simulink model "rlDDPG4PFC2"  (R2022b)
settings: Solver=FixedStepAuto  StartTime=0.0  StopTime=Tf  FixedStep=0.001  RelTol=1e-3
StartFcn:
  | %scopes= find_system(bdroot,'BlockType','Scope');
  | %for i = 1:length(scopes)
  | %set_param(scopes{i},'Open','on');
  | %end
values from neighbouring files (symbols this model uses):
  amax_ego = 0.4    [DDPG_1.m]    (also in DQN4.m)
  amin_ego = -0.5    [DDPG_1.m]    (also in DQN4.m)
  Cf = 19000    [DDPG_1.m]    (also in DQN4.m)
  Cr = 33000    [DDPG_1.m]    (also in DQN4.m)
  D_default = 1.5    [DDPG_1.m]    (also in DQN4.m)
  e1_initial = -0.05    [DDPG_1.m]    (also in DQN4.m)
  e2_initial = 0.05    [DDPG_1.m]    (also in DQN4.m)
  Iz = 2875    [DDPG_1.m]    (also in DQN4.m)
  lf = 1.4    [DDPG_1.m]    (also in DQN4.m)
  lr = 1.6    [DDPG_1.m]    (also in DQN4.m)
  m = 1600    [DDPG_1.m]    (also in DQN4.m)
  t_gap = 1.4    [DDPG_1.m]    (also in DQN4.m)
  target = 1    [DDPG_1.m]    (also in DQN4.m = 3)
  tau = 0.5    [DDPG_1.m]    (also in DQN4.m)
  Ts = 0.1    [DDPG_1.m]    (also in DQN4.m)
  umax_ego = 0.2618    [DDPG_1.m]    (also in DQN4.m)
  umin_ego = -0.2618    [DDPG_1.m]    (also in DQN4.m)
  v0_FV1 = 0.5    [DDPG_1.m]    (also in DQN4.m)
  v0_FV2 = 0.5    [DDPG_1.m]    (also in DQN4.m)
  v0_LV = 0.9    [DDPG_1.m]    (also in DQN4.m)
  v_set = 1.5    [DDPG_1.m]    (also in DQN4.m)
  x0_FV1 = 1.5    [DDPG_1.m]    (also in DQN4.m)
  x0_FV2 = 0    [DDPG_1.m]    (also in DQN4.m)
  x0_LV = 3    [DDPG_1.m]    (also in DQN4.m)
undefined symbols (not defined in the file or in its folder): DiscIntNeverNeededParam, Speed, SteeringAngle
libraries: simulink x19, rllib x4, robotlib x4, dsparch4 x2
(part 2 of 2)

== system rlDDPG4PFC2/Ego Vehicle and Environment3/Lead vehicle1/ramp1 ==
  note: 工况1：斜坡加速度
  Clock : Clock
  Constant1 : Constant  Value=20
  Constant2 : Constant  Value=40
  Ramp : simulink/Sources/Ramp  slope=0.001  start=0  InitialOutput=0
  Ramp1 : simulink/Sources/Ramp  slope=-0.001  start=20  InitialOutput=0.02
  Ramp2 : simulink/Sources/Ramp  slope=0  start=40  InitialOutput=0
  Relational Operator : RelationalOperator  Operator=<=  OutDataTypeStr=boolean  RndMeth=Simplest  InputSameDT=off
  Relational Operator1 : RelationalOperator  Operator=<=  OutDataTypeStr=boolean  RndMeth=Simplest  InputSameDT=off
  Switch : Switch  Criteria=u2 > Threshold  SaturateOnIntegerOverflow=off  InputSameDT=off
  Switch1 : Switch  Criteria=u2 > Threshold  SaturateOnIntegerOverflow=off  InputSameDT=off
  Out1 : Outport
  wires:
  Constant1/1 -> Relational Operator/2
  Ramp1/1 -> Switch1/1
  Relational Operator/1 -> Switch/2
  Switch1/1 -> Switch/3
  Relational Operator1/1 -> Switch1/2
  Clock/1 -> Relational Operator1/1, Relational Operator/1
  Ramp/1 -> Switch/1
  Constant2/1 -> Relational Operator1/2
  Ramp2/1 -> Switch1/3
  Switch/1 -> Out1/1

== system rlDDPG4PFC2/Ego Vehicle and Environment3/Lead vehicle1/step1 ==
  note: 工况3：阶梯式加速-减速
  Add : Sum  Inputs=++++
  Step : Step  Time=5  After=0.2  SampleTime=0
  Step1 : Step  Time=8  After=-0.2  SampleTime=0
  Step2 : Step  Time=40  After=-0.2  SampleTime=0
  Step3 : Step  Time=43  After=0.2  SampleTime=0
  a_LV : Outport
  wires:
  Step2/1 -> Add/3
  Step3/1 -> Add/4
  Step/1 -> Add/1
  Add/1 -> a_LV/1  "a_LV"
  Step1/1 -> Add/2

== matlab function rlDDPG4PFC2/Ego Vehicle and Environment1/curvature1/N-curve ==
  data: s input; rho output
function rho = fcn(s)
% 根据输入s计算输出rho
if s >= 0 && s < 5
  rho = 0;
elseif s >= 5 && s < 10
  rho = 0.025*4;
elseif s >= 10 && s < 30
  rho = -0.025;
elseif s >= 30 && s < 40
  rho = -0.0855;
elseif s >= 40 && s < 60
  rho = 0.057;
else  % s >= 60
  rho = 0;
end

== matlab function rlDDPG4PFC2/Ego Vehicle and Environment1/curvature1/S-curve ==
  data: s input; rho output
function rho = fcn(s)
% 根据输入s计算输出rho
if s >= 0 && s < 10
  rho = 0;
elseif s >= 10 && s < 40
  rho = 0.005*4;
elseif s >= 40 && s < 70
  rho = -0.005*4;
else  % s >= 70
  rho = 0;
end

== matlab function rlDDPG4PFC2/Ego Vehicle and Environment3/curvature1/M-curve ==
  data: s input; rho output
function rho = fcn(s)
% 根据输入s计算输出rho
if s >= 0 && s < 5
  rho = 0;
elseif s >= 5 && s < 13
  rho = 0.1;
elseif s >= 13 && s < 25
  rho = -0.0667;
elseif s >= 25 && s < 27
  rho = 0;
elseif s >= 27 && s < 33
  rho = -0.05;
elseif s >= 33 && s < 53
  rho = 0.03;
elseif s >= 53 && s < 59
    rho = -0.05;
elseif s >= 59 && s < 61
    rho = 0;
elseif s >= 61 && s < 73
  rho = -0.0667;
elseif s >= 73 && s < 81
  rho = 0.1;
else  % s >= 70
  rho = 0;
end

== matlab function rlDDPG4PFC2/Ego Vehicle and Environment3/curvature1/N-curve ==
  data: s input; rho output
function rho = fcn(s)
% 根据输入s计算输出rho
if s >= 0 && s < 5
  rho = 0;
elseif s >= 5 && s < 10
  rho = 0.025*4;
elseif s >= 10 && s < 30
  rho = -0.025;
elseif s >= 30 && s < 40
  rho = -0.0855;
elseif s >= 40 && s < 60
  rho = 0.057;
else  % s >= 60
  rho = 0;
end

== matlab function rlDDPG4PFC2/Ego Vehicle and Environment3/curvature1/S-curve ==
  data: s input; rho output
function rho = fcn(s)
% 根据输入s计算输出rho
if s >= 0 && s < 10
  rho = 0;
elseif s >= 10 && s < 40
  rho = 0.005*4;
elseif s >= 40 && s < 70
  rho = -0.005*4;
else  % s >= 70
  rho = 0;
end

== matlab function rlDDPG4PFC2/Ego Vehicle and Environment1/curvature1/M-curve ==
  data: s input; rho output
function rho = fcn(s)
% 根据输入s计算输出rho
if s >= 0 && s < 5
  rho = 0;
elseif s >= 5 && s < 13
  rho = 0.1;
elseif s >= 13 && s < 25
  rho = -0.0667;
elseif s >= 25 && s < 27
  rho = 0;
elseif s >= 27 && s < 33
  rho = -0.05;
elseif s >= 33 && s < 53
  rho = 0.03;
elseif s >= 53 && s < 59
    rho = -0.05;
elseif s >= 59 && s < 61
    rho = 0;
elseif s >= 61 && s < 73
  rho = -0.0667;
elseif s >= 73 && s < 81
  rho = 0.1;
else  % s >= 70
  rho = 0;
end
